simulink model "Inv_Pend"  (R2019b)
settings: Solver=FixedStepAuto  StartTime=0.0  StopTime=6  FixedStep=0.01  RelTol=1e-3
settings Model: Creator=cambr  LastModifiedBy=cambr

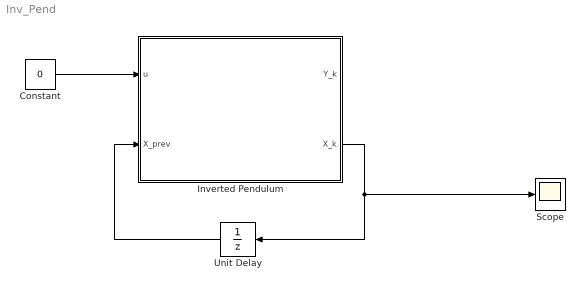
== system Inv_Pend ==
  Constant : Constant  Value=0
  Inverted Pendulum : MATLAB Function  TreatAsAtomicUnit=on
  Scope : Scope
  Unit Delay : UnitDelay  InitialCondition=[0; 0; 0.01; 0]  SampleTime=-1  HasFrameUpgradeWarning=on
  wires:
  Inverted Pendulum/2(X_k) -> Unit Delay/1, Scope/1
  Unit Delay/1 -> Inverted Pendulum/2(X_prev)
  Constant/1 -> Inverted Pendulum/1(u)

== matlab function Inv_Pend/Inverted Pendulum ==
  data: u input; Y_k output; X_prev input; X_k output
function [Y_k, X_k] = fcn(u, X_prev)
%% Discrete Matrices
Ad = [1.0000 0.0100    0      0;
          0  0.9997 0.0085 0.0000;
          0 -0.0000 1.0012 0.0100;
          0 -0.0006 0.2492 1.0012];
Bd = [0.0001;
      0.0274;
      0.0636;
      0.0079];
 
Cd = [1 0 0 0;
      0 0 1 0];
  
%% State Equation  
X_k = Ad*X_prev + Bd*u;

%% Measurement Equation
Y_k = Cd*X_k;
